simulink model "firstbpsk6"  (Simulink 9.1)
settings: Solver=FixedStepDiscrete  StartTime=0.0  StopTime=500  RelTol=1e-3  EnableMultiTasking=on
libraries: dsp_blocks x5
settings Model: Creator=DSP_Lab  LastModifiedBy=Hayoung
settings DataIOCC: LimitDataPoints=on
settings OptimizationCC: ExpressionDepthLimit=2147483647
settings DebuggingCC: SolverPrmCheckMsg=warning  StateNameClashWarn=warning
settings GRTTargetCC: GeneratePreprocessorConditionals=Disable all  CombineOutputUpdateFcns=on  GRTInterface=off

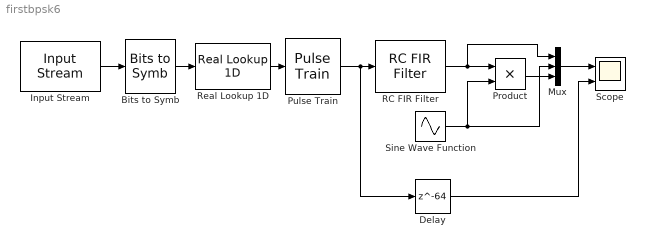
== system firstbpsk6 ==
  Bits to Symb : dsp_blocks/Conversions/Bits to Symb
  Delay : Delay  DelayLength=64
  Input Stream : dsp_blocks/Sources//Sinks/Input Stream  period=50  width=1  fname=rand.mat
  Mux : Mux  Inputs=3
  Product : Product  RndMeth=Zero
  Pulse Train : dsp_blocks/Conversions/Pulse Train  period=50
  RC FIR Filter : dsp_blocks/Filters/RC FIR Filter  period=50  beta=0.25  root=off  filt_len=128  win_type=on
  Real Lookup 1D : dsp_blocks/Conversions/Real Lookup 1D  table=[-1 1]
  Scope : Scope  NumInputPorts=2
  Sine Wave Function : Sin  Frequency=2*pi*0.1  SampleTime=0
  wires:
  Input Stream/1 -> Bits to Symb/1
  Bits to Symb/1 -> Real Lookup 1D/1
  Pulse Train/1 -> Delay/1, RC FIR Filter/1
  Real Lookup 1D/1 -> Pulse Train/1
  RC FIR Filter/1 -> Mux/1, Product/1
  Sine Wave Function/1 -> Mux/2, Product/2
  Product/1 -> Mux/3
  Mux/1 -> Scope/1
  Delay/1 -> Scope/2
